simulink model "coupled_tanks_quick_start"  (Simulink 8.3)
settings: Solver=ode1  StartTime=0.0  StopTime=inf  FixedStep=0.1  RelTol=1e-3
PostLoadFcn:
  | qc_set_target_type(getConfigSet(bdroot, 'QUARC Default Target Configuration'));
undefined symbols (not defined in the file or in its folder): HIL
libraries: quarc_library x3
settings Model: Creator=MLevis  LastModifiedBy=Aluno IC  SimulationMode=external  ExtModeTrigDuration=30000
settings SolverCC: PositivePriorityOrder=on
settings OptimizationCC: ExpressionDepthLimit=2147483647  InitFltsAndDblsToZero=on
settings DebuggingCC: SaveWithParameterizedLinksMsg=none  MultiTaskDSMMsg=warning  MultiTaskCondExecSysMsg=none  FcnCallInpInsideContextMsg=UseLocalSettings
settings RTWCC: SystemTargetFile=quarc_win64.tlc  TemplateMakefile=quarc_default_tmf  Description=QUARC Win64 Target  ProcessScript=quarc_win64_make_rtw_hook
settings STFCustomTargetCC: TargetPreCompLibLocation=C:\PROGRA~3\QUARC\lib\2014a\win64\release  ConcurrentExecutionCompliant=on  GeneratePreprocessorConditionals=Disable all  CPPClassGenCompliant=on  SystemTargetFile=quarc_win64.tlc
settings GRTTargetCC: TargetPreCompLibLocation=C:\PROGRA~3\QUARC\lib\2014a\win64\release  ParMdlRefBuildCompliant=off  CompOptLevelCompliant=off  MatFileLogging=off  ExtMode=on  ExtModeMexFile=quarc_comm

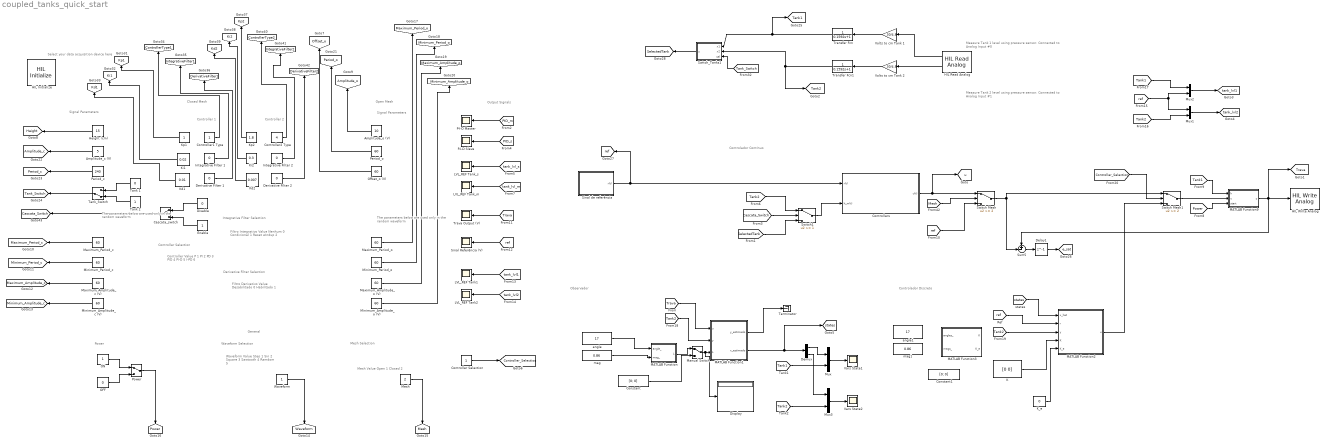
== system coupled_tanks_quick_start ==
  note: Controlador Discreto
  note: Observador
  note: Controlador Contínuo
  note: Measure Tank 2 level using pressure sensor.
      | Connected to Analog Input #1
  note: Measure Tank 1 level using pressure sensor.
      | Connected to Analog Input #0
  note: Select your data acquisition device here
  note: Output Signals
  note: Controller
      | Value
      |
      | P
      | 1
      |
      | PI
      | 2
      |
      | PD
      | 3
      |
      | PID
      | 4
      |
      | PI-D
      | 5
      |
      | I-PD
      | 6
  note: Controller Selection
  note: Signal Parameters
  note: Mesh
      | Value
      |
      | Open
      | 1
      |
      | Closed
      | 2
  note: Mesh Selection
  note: Power
  note: Waveform
      | Value
      |
      | Step
      | 1
      |
      | Sin
      | 2
      |
      | Square
      | 3
      |
      | Sawtooth
      | 4
      |
      | Ramdom
      | 5
  note: Waveform Selection
  note: General
  note: Controller 1
  note: The parameters below are used only in the random waveform
  note: Signal Parameters
  note: The parameters below are used only in the random waveform
  note: Open Mesh
  note: Controller 2
  note: Filtro Derivativo
      | Value
      |
      | Desabilitado
      | 0
      |
      | Habilitado
      | 1
  note: Filtro Integrativo
      | Value
      |
      | Nenhum
      | 0
      |
      | Condicional
      | 1
      |
      | Reset windup
      | 2
  note: Integrative Filter Selection
  note: Derivative Filter Selection
  note: Closed Mesh
  Amplitude_c (V) : Constant  Value=5
  Amplitude_o (V) : Constant  Value=10
  Cascata_switch : ManualSwitch
  Constant : Constant  Value=[0; 0]
  Constant1 : Constant  Value=[0; 0]
  Controller Selection : Constant
  Controller1 Type : Constant
  Controller2 Type : Constant  Value=4
  Controllers : Subsystem
  Delay1 : Delay  DelayLength=1  InitialCondition=0
  Demux : Demux  Outputs=2
  Derivative Filter 1 : Constant  Value=0
  Derivative Filter 2 : Constant  Value=0
  Disable : Constant  Value=0
  Display : Display
  Enable : Constant
  HIL Initialize : quarc_library/Data Acquisition/Generic/Configuration/HIL Initialize  object_name=HIL-1  board_type=q2_usb  board_number=0  board_options=d0=digital;d1=digital;led=auto;update_rate=normal;decimation=1  exclusive=off  active=off  hardware_clocks=[0]  clock_modes=[]  initial_clock_frequencies=[]  set_clock_params_at_start=off  set_clock_params_at_switch_in=off  set_clock_frequencies_at_start=off  set_clock_frequencies_at_switch_in=off  analog_input_channels=[0:1]  analog_input_maximums=10  analog_input_minimums=-10  set_analog_input_params_at_start=on  set_analog_input_params_at_switch_in=off  analog_output_channels=[0:1]  analog_output_maximums=10  analog_output_minimums=-10  initial_analog_outputs=[0]  final_analog_outputs=[0]  watchdog_analog_outputs=0  set_analog_output_params_at_start=on  set_analog_output_params_at_switch_in=off  set_analog_outputs_at_start=on  set_analog_outputs_at_switch_in=off  set_analog_outputs_at_terminate=on  set_analog_outputs_at_switch_out=off  set_analog_outputs_on_watchdog=off  digital_input_channels=[]  digital_output_channels=[]  digital_output_configuration=[]  initial_digital_outputs=[1]  final_digital_outputs=[1]  watchdog_digital_outputs=[1]  set_digital_output_params_at_start=off  set_digital_output_params_at_switch_in=off  set_digital_outputs_at_start=on  set_digital_outputs_at_switch_in=off  set_digital_outputs_at_terminate=on  set_digital_outputs_at_switch_out=off  set_digital_outputs_on_watchdog=off  encoder_channels=[0:1]  quadrature=[4]  encoder_filter_frequency=[]  initial_encoder_counts=[0]  set_encoder_params_at_start=on  set_encoder_params_at_switch_in=off  set_encoder_counts_at_start=on  set_encoder_counts_at_switch_in=off  pwm_channels=[]  pwm_modes=[0]  pwm_frequency=1/0.020  pwm_configuration=[]  pwm_alignment=[]  pwm_polarity=[]  pwm_leading_deadband=[]  pwm_trailing_deadband=[]  initial_pwm_outputs=[0]  final_pwm_outputs=[0]  watchdog_pwm_outputs=[0]  set_pwm_params_at_start=on  set_pwm_params_at_switch_in=off  set_pwm_outputs_at_start=on  set_pwm_outputs_at_switch_in=off  set_pwm_outputs_at_terminate=on  set_pwm_outputs_at_switch_out=off  set_pwm_outputs_on_watchdog=off  other_output_channels=[]  initial_other_outputs=[]  final_other_outputs=[]  watchdog_other_outputs=[]  set_other_outputs_at_start=off  set_other_outputs_at_switch_in=off  set_other_outputs_at_terminate=off  set_other_outputs_at_switch_out=off  set_other_outputs_on_watchdog=off
  HIL Read Analog : quarc_library/Data Acquisition/Generic/Immediate I//O/HIL Read Analog  object_name=HIL-1  channels=[0:1]  sample_time=qc_get_step_size  active=on  vector_output=off
  HIL Write Analog : quarc_library/Data Acquisition/Generic/Immediate I//O/HIL Write Analog  object_name=HIL-1  channels=0  sample_time=-1  active=off  vector_input=off
  Height (cm) : Constant  Value=15
  Integrative Filter 1 : Constant  Value=0
  Integrative Filter 2 : Constant  Value=0
  K : Constant  Value=[0 0]  VectorParams1D=off
  K_e : Constant  Value=0  VectorParams1D=off
  Kd1 : Constant  Value=0.01
  Kd2 : Constant  Value=0.007
  Ki1 : Constant  Value=0.02
  Ki2 : Constant  Value=0.3
  Kp1 : Constant
  Kp2 : Constant  Value=1.8
  LVL_REF Tank1 : Scope
      settings: ShowLegends=on  TimeRange=100  YMin=0  YMax=30  SaveName=tank1level1
  LVL_REF Tank2 : Scope
      settings: ShowLegends=on  TimeRange=250  YMin=0  YMax=30  SaveName=tank2level1
  "LVL_REF Tank_m " : Scope
      settings: ShowLegends=on  TimeRange=300  YMin=0  YMax=30  SaveName=tank2level
  LVL_REF Tank_s : Scope
      settings: ShowLegends=on  TimeRange=300  YMin=-90  YMax=130  SaveName=tank1level
  MATLAB Function : MATLAB Function  TreatAsAtomicUnit=on
  MATLAB Function1 : MATLAB Function  TreatAsAtomicUnit=on
  MATLAB Function2 : MATLAB Function  TreatAsAtomicUnit=on
  MATLAB Function3 : MATLAB Function  TreatAsAtomicUnit=on
  MATLAB Function9 : MATLAB Function  TreatAsAtomicUnit=on
  Manual Switch : ManualSwitch
  Maximum_Amplitude_c (V) : Constant  Value=60
  Maximum_Amplitude_o (V) : Constant  Value=60
  Maximum_Period_c : Constant  Value=60
  Maximum_Period_o : Constant  Value=60
  Mesh : Constant  Value=2
  Minimum_Amplitude_c (V) : Constant  Value=60
  Minimum_Amplitude_o (V) : Constant  Value=60
  Minimum_Period_c : Constant  Value=60
  Minimum_Period_o : Constant  Value=60
  Mux{,1..3} (4 alike) : Mux  Inputs=2
  OFF : Constant  Value=0
  ON : Constant
  Offset_o (V) : Constant  Value=60
  P-I-D Master : Scope
      settings: ShowLegends=on  TimeRange=300  YMin=-35  YMax=30  SaveName=PID1
  P-I-D Slave : Scope
      settings: ShowLegends=on  TimeRange=300  YMin=-35  YMax=80  SaveName=PID2
  Period_c : Constant  Value=240
  Period_o : Constant  Value=60
  Power : ManualSwitch
  Sinal Referência (V) : Scope
      settings: TimeRange=300  YMin=0  YMax=30  SaveName=meshoutput
  Sinal de referência : Subsystem
  Sum5 : Sum  Inputs=+-|
  Switch Mesh : Switch  Threshold=2
  Switch Mesh1 : Switch  Threshold=2
  Switch1 : Switch  Threshold=1
  Switch_Tanks1 : MATLAB Function  TreatAsAtomicUnit=on
  Tank 1 : Constant  Value=0
  Tank 2 : Constant
  Tank_Switch : ManualSwitch  CurrentSetting=0
  Terminator : Terminator
  Transfer Fcn : TransferFcn  Denominator=[0.1592 1]
  Transfer Fcn1 : TransferFcn  Denominator=[0.1592 1]
  Trava Output (V) : Scope
      settings: TimeRange=300  YMin=-4.5  YMax=4.5  SaveName=meshoutput2
  Vars State1 : Scope
      settings: ShowLegends=on  TimeRange=100  YMin=-1  YMax=30  SaveName=state1
  Vars State2 : Scope
      settings: ShowLegends=on  TimeRange=100  YMin=-1  YMax=30  SaveName=state2
  "Volts to cm Tank 1 " : Gain  Gain=30/4.8
  Volts to cm Tank 2 : Gain  Gain=30/4.8
  Waveform : Constant
  angle : Constant  Value=17
  angle1 : Constant  Value=17
  mag : Constant  Value=0.86
  mag1 : Constant  Value=0.86
  tag scope: Amplitude_c=global, Amplitude_o=global, Cascata_Switch=global, ControllerType1=global, ControllerType2=global, Controller_Selection=global, DerivativeFilter1=global, DerivativeFilter2=global, Height=global, IntegrativeFilter1=global, IntegrativeFilter2=global, Kd1=global, Kd2=global, Ki1=global, Ki2=global, Kp1=global, Kp2=global, Maximum_Amplitude_c=global, Maximum_Amplitude_o=global, Maximum_Period_c=global, Maximum_Period_o=global, Mesh=global, Minimum_Amplitude_c=global, Minimum_Amplitude_o=global, Minimum_Period_c=global, Minimum_Period_o=global, Offset_o=global, Period_c=global, Period_o=global, Power=global, SelectedTank=global, Tank1=global, Tank2=global, Tank_Switch=global, Trava=global, Waveform=global, e_sat=global, ref=global, states=global, tank_lvl1=global, tank_lvl2=global, u=global
  wires:
  HIL Read Analog/1 -> "Volts to cm Tank 1 "/1
  "Volts to cm Tank 1 "/1 -> Transfer Fcn/1
  Volts to cm Tank 2/1 -> Transfer Fcn1/1
  HIL Read Analog/2 -> Volts to cm Tank 2/1
  [Cascata_Switch] -> Switch1/2
  [SelectedTank] -> Switch1/3
  [Tank2] -> Switch1/1
  ON/1 -> Power/1
  OFF/1 -> Power/2
  Tank 1/1 -> Tank_Switch/1
  Tank 2/1 -> Tank_Switch/2
  Height (cm)/1 -> [Height]
  Tank_Switch/1 -> [Tank_Switch]
  Amplitude_c (V)/1 -> [Amplitude_c]
  Period_c/1 -> [Period_c]
  Maximum_Period_c/1 -> [Maximum_Period_c]
  Minimum_Period_c/1 -> [Minimum_Period_c]
  Maximum_Amplitude_c (V)/1 -> [Maximum_Amplitude_c]
  Minimum_Amplitude_c (V)/1 -> [Minimum_Amplitude_c]
  Waveform/1 -> [Waveform]
  Mesh/1 -> [Mesh]
  Power/1 -> [Power]
  Amplitude_o (V)/1 -> [Amplitude_o]
  Period_o/1 -> [Period_o]
  Offset_o (V)/1 -> [Offset_o]
  Maximum_Period_o/1 -> [Maximum_Period_o]
  Minimum_Period_o/1 -> [Minimum_Period_o]
  Maximum_Amplitude_o (V)/1 -> [Maximum_Amplitude_o]
  Minimum_Amplitude_o (V)/1 -> [Minimum_Amplitude_o]
  Kp1/1 -> [Kp1]
  Ki1/1 -> [Ki1]
  Kd1/1 -> [Kd1]
  Controller1 Type/1 -> [ControllerType1]
  Integrative Filter 1/1 -> [IntegrativeFilter1]
  Derivative Filter 1/1 -> [DerivativeFilter1]
  Kp2/1 -> [Kp2]
  Ki2/1 -> [Ki2]
  Kd2/1 -> [Kd2]
  Derivative Filter 2/1 -> [DerivativeFilter2]
  Integrative Filter 2/1 -> [IntegrativeFilter2]
  Controller2 Type/1 -> [ControllerType2]
  Disable/1 -> Cascata_switch/1
  Enable/1 -> Cascata_switch/2
  Cascata_switch/1 -> [Cascata_Switch]
  Switch Mesh/1 -> Switch Mesh1/1, Sum5/2
  [Tank1] -> MATLAB Function9/1(h)
  [Mesh] -> Switch Mesh/2
  Switch_Tanks1/1(y) -> [SelectedTank]
  Sinal de referência/1(r(t)) -> Controllers/1(r(t)), [ref]
  [Tank_Switch] -> Switch_Tanks1/3(sel)
  Transfer Fcn1/1 -> Switch_Tanks1/2(x2), [Tank2]
  Transfer Fcn/1 -> Switch_Tanks1/1(x1), [Tank1]
  [Power] -> MATLAB Function9/3(start)
  Controllers/1(u(t)) -> [u], Switch Mesh/1
  MATLAB Function9/1(y) -> [Trava], Sum5/1, HIL Write Analog/1
  Delay1/1 -> [e_sat]
  Sum5/1 -> Delay1/1
  [ref] -> Switch Mesh/3
  Switch1/1 -> Controllers/2(h_m(t))
  [PID_m] -> P-I-D Master/1
  [PID_s] -> P-I-D Slave/1
  [tank_lvl_m] -> "LVL_REF Tank_m "/1
  [tank_lvl_s] -> LVL_REF Tank_s/1
  [Trava] -> Trava Output (V)/1
  [ref] -> Sinal Referência (V)/1
  [Tank1] -> Mux2/1
  [ref] -> Mux2/2, Mux1/1
  [Tank2] -> Mux1/2
  Mux2/1 -> [tank_lvl1]
  Mux1/1 -> [tank_lvl2]
  [tank_lvl1] -> LVL_REF Tank1/1
  [tank_lvl2] -> LVL_REF Tank2/1
  mag/1 -> MATLAB Function/2(mag_)
  angle/1 -> MATLAB Function/1(angle_)
  [Trava] -> MATLAB Function1/1(u)
  [Tank2] -> MATLAB Function1/2(y)
  MATLAB Function1/2(x_estimado) -> [states], Demux/1
  Mux/1 -> Vars State1/1
  [Tank1] -> Mux/2
  Constant/1 -> Manual Switch/2
  Demux/1 -> Mux/1
  Demux/2 -> Mux3/1
  [Tank2] -> Mux3/2
  Mux3/1 -> Vars State2/1
  Manual Switch/1 -> Display/1, MATLAB Function1/3(L)
  MATLAB Function/1(L) -> Manual Switch/1
  MATLAB Function1/1(y_estimado) -> Terminator/1
  [states] -> MATLAB Function2/1(x_hat)
  [ref] -> MATLAB Function2/2(r)
  [Tank2] -> MATLAB Function2/3(y)
  K/1 -> MATLAB Function2/4(K)
  K_e/1 -> MATLAB Function2/5(K_e)
  Switch Mesh1/1 -> MATLAB Function9/2(u)
  MATLAB Function2/1(u) -> Switch Mesh1/3
  [Controller_Selection] -> Switch Mesh1/2
  Controller Selection/1 -> [Controller_Selection]

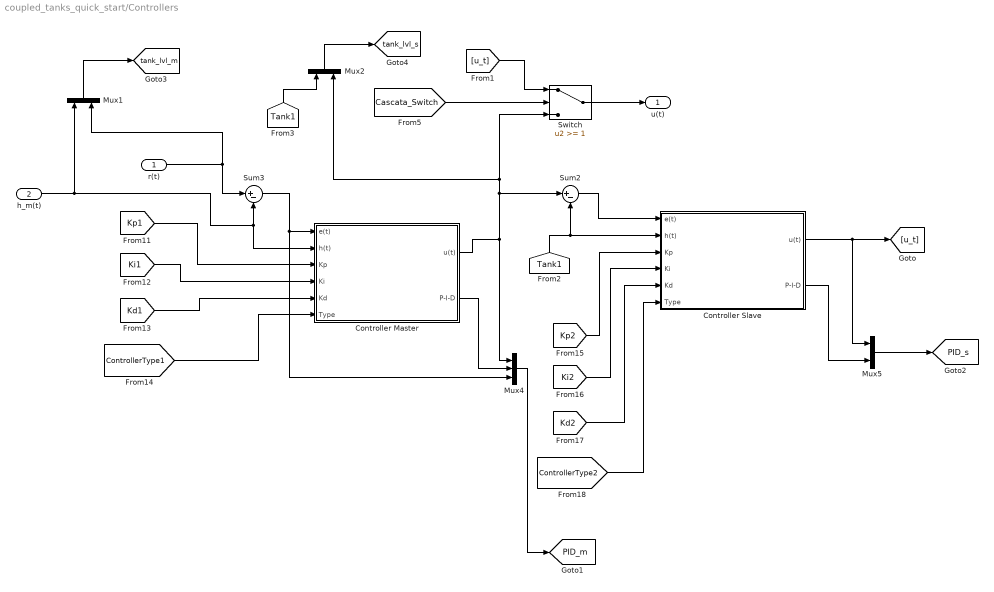
== system coupled_tanks_quick_start/Controllers ==
  r(t) : Inport
  h_m(t) : Inport  Port=2
  Controller Master : Subsystem
  Controller Slave : Subsystem
  Mux1 : Mux  Inputs=2
  Mux2 : Mux  Inputs=2
  Mux4 : Mux  Inputs=3
  Mux5 : Mux  Inputs=2
  Sum2 : Sum  Inputs=|+-
  Sum3 : Sum  Inputs=|+-
  Switch : Switch  Threshold=1
  u(t) : Outport
  tag scope: PID_m=global, PID_s=global, tank_lvl_m=global, tank_lvl_s=global
  wires:
  [Tank1] -> Controller Slave/2(h(t)), Sum2/2
  [Kd1] -> Controller Master/5(Kd)
  Controller Slave/2(P-I-D) -> Mux5/2
  [Kp2] -> Controller Slave/3(Kp)
  [Ki2] -> Controller Slave/4(Ki)
  [Ki1] -> Controller Master/4(Ki)
  [Kd2] -> Controller Slave/5(Kd)
  [ControllerType2] -> Controller Slave/6(Type)
  [Kp1] -> Controller Master/3(Kp)
  [ControllerType1] -> Controller Master/6(Type)
  h_m(t)/1 -> Sum3/2, Controller Master/2(h(t)), Mux1/1
  Controller Master/1(u(t)) -> Mux2/2, Switch/3, Sum2/1, Mux4/1
  Sum2/1 -> Controller Slave/1(e(t))
  Controller Slave/1(u(t)) -> [u_t], Mux5/1
  r(t)/1 -> Sum3/1, Mux1/2
  Switch/1 -> u(t)/1
  [Cascata_Switch] -> Switch/2
  Sum3/1 -> Mux4/3, Controller Master/1(e(t))
  [u_t] -> Switch/1
  Mux1/1 -> [tank_lvl_m]
  [Tank1] -> Mux2/1
  Mux2/1 -> [tank_lvl_s]
  Mux4/1 -> [PID_m]
  Mux5/1 -> [PID_s]
  Controller Master/2(P-I-D) -> Mux4/2

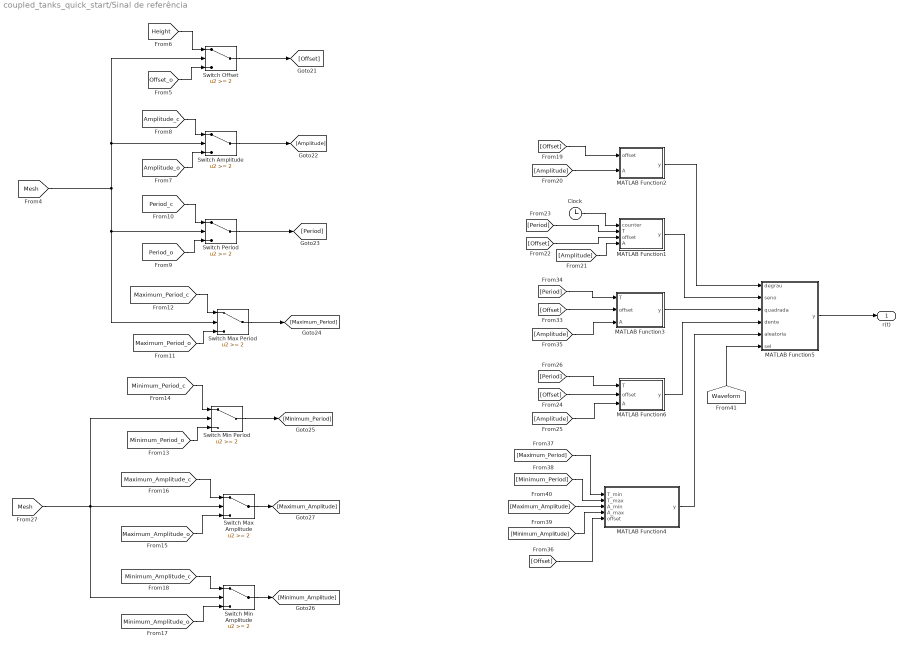
== system coupled_tanks_quick_start/Sinal de referência ==
  Clock : Clock
  MATLAB Function1 : MATLAB Function  TreatAsAtomicUnit=on
  MATLAB Function2 : MATLAB Function  TreatAsAtomicUnit=on
  MATLAB Function3 : MATLAB Function  TreatAsAtomicUnit=on
  MATLAB Function4 : MATLAB Function  TreatAsAtomicUnit=on
  MATLAB Function5 : MATLAB Function  TreatAsAtomicUnit=on
  MATLAB Function6 : MATLAB Function  TreatAsAtomicUnit=on
  Switch Amplitude : Switch  Threshold=2
  Switch Max Amplitude : Switch  Threshold=2
  Switch Max Period : Switch  Threshold=2
  Switch Min Amplitude : Switch  Threshold=2
  Switch Min Period : Switch  Threshold=2
  Switch Offset : Switch  Threshold=2
  Switch Period : Switch  Threshold=2
  r(t) : Outport
  wires:
  Clock/1 -> MATLAB Function1/1(counter)
  MATLAB Function5/1(y) -> r(t)/1
  [Mesh] -> Switch Max Period/2, Switch Period/2, Switch Offset/2, Switch Amplitude/2
  [Offset] -> MATLAB Function6/2(offset)
  Switch Min Amplitude/1 -> [Minimum_Amplitude]
  [Period] -> MATLAB Function6/1(T)
  Switch Amplitude/1 -> [Amplitude]
  Switch Period/1 -> [Period]
  Switch Offset/1 -> [Offset]
  [Amplitude] -> MATLAB Function2/2(A)
  Switch Min Period/1 -> [Minimum_Period]
  [Amplitude] -> MATLAB Function1/4(A)
  Switch Max Amplitude/1 -> [Maximum_Amplitude]
  Switch Max Period/1 -> [Maximum_Period]
  [Offset] -> MATLAB Function1/3(offset)
  [Offset] -> MATLAB Function2/1(offset)
  [Period] -> MATLAB Function1/2(T)
  [Amplitude] -> MATLAB Function6/3(A)
  [Period] -> MATLAB Function3/1(T)
  MATLAB Function1/1(y) -> MATLAB Function5/2(seno)
  [Waveform] -> MATLAB Function5/6(sel)
  [Maximum_Period] -> MATLAB Function4/1(T_min)
  [Mesh] -> Switch Min Amplitude/2, Switch Max Amplitude/2, Switch Min Period/2
  MATLAB Function2/1(y) -> MATLAB Function5/1(degrau)
  [Maximum_Amplitude] -> MATLAB Function4/3(A_min)
  MATLAB Function6/1(y) -> MATLAB Function5/4(dente)
  [Amplitude] -> MATLAB Function3/3(A)
  [Minimum_Amplitude] -> MATLAB Function4/4(A_max)
  [Offset] -> MATLAB Function4/5(offset)
  MATLAB Function4/1(y) -> MATLAB Function5/5(aleatoria)
  MATLAB Function3/1(y) -> MATLAB Function5/3(quadrada)
  [Offset] -> MATLAB Function3/2(offset)
  [Minimum_Period] -> MATLAB Function4/2(T_max)
  [Offset_o] -> Switch Offset/3
  [Height] -> Switch Offset/1
  [Amplitude_o] -> Switch Amplitude/3
  [Amplitude_c] -> Switch Amplitude/1
  [Period_o] -> Switch Period/3
  [Period_c] -> Switch Period/1
  [Maximum_Period_o] -> Switch Max Period/3
  [Maximum_Period_c] -> Switch Max Period/1
  [Minimum_Period_c] -> Switch Min Period/1
  [Minimum_Period_o] -> Switch Min Period/3
  [Maximum_Amplitude_c] -> Switch Max Amplitude/1
  [Maximum_Amplitude_o] -> Switch Max Amplitude/3
  [Minimum_Amplitude_c] -> Switch Min Amplitude/1
  [Minimum_Amplitude_o] -> Switch Min Amplitude/3

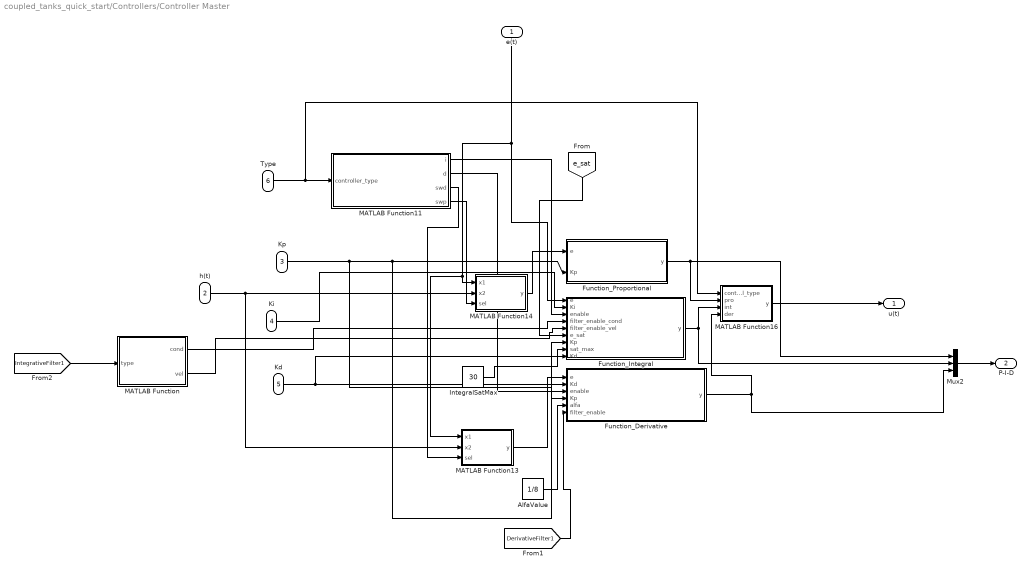
== system coupled_tanks_quick_start/Controllers/Controller Master ==
  e(t) : Inport
  h(t) : Inport  Port=2
  Kp : Inport  Port=3
  Ki : Inport  Port=4
  Kd : Inport  Port=5
  Type : Inport  Port=6
  AlfaValue : Constant  Value=1/8
  Function_Derivative : MATLAB Function  TreatAsAtomicUnit=on
  Function_Integral : MATLAB Function  TreatAsAtomicUnit=on
  Function_Proportional : MATLAB Function  TreatAsAtomicUnit=on
  IntegralSatMax : Constant  Value=30
  MATLAB Function : MATLAB Function  TreatAsAtomicUnit=on
  MATLAB Function11 : MATLAB Function  TreatAsAtomicUnit=on
  MATLAB Function13 : MATLAB Function  TreatAsAtomicUnit=on
  MATLAB Function14 : MATLAB Function  TreatAsAtomicUnit=on
  MATLAB Function16 : MATLAB Function  TreatAsAtomicUnit=on
  Mux2 : Mux  Inputs=3
  u(t) : Outport
  P-I-D : Outport  Port=2
  wires:
  h(t)/1 -> MATLAB Function13/2(x2), MATLAB Function14/2(x2)
  e(t)/1 -> MATLAB Function13/1(x1), MATLAB Function14/1(x1), Function_Integral/1(e)
  Function_Integral/1(y) -> MATLAB Function16/3(int), Mux2/2
  Kp/1 -> Function_Derivative/4(Kp), Function_Integral/7(Kp), Function_Proportional/2(Kp)
  MATLAB Function11/2(d) -> Function_Derivative/3(enable)
  Function_Proportional/1(y) -> MATLAB Function16/2(pro), Mux2/1
  MATLAB Function11/1(i) -> Function_Integral/3(enable)
  Type/1 -> MATLAB Function16/1(control_type), MATLAB Function11/1(controller_type)
  MATLAB Function11/4(swp) -> MATLAB Function14/3(sel)
  Ki/1 -> Function_Integral/2(Ki)
  MATLAB Function/2(vel) -> Function_Integral/5(filter_enable_vel)
  MATLAB Function11/3(swd) -> MATLAB Function13/3(sel)
  MATLAB Function/1(cond) -> Function_Integral/4(filter_enable_cond)
  IntegralSatMax/1 -> Function_Integral/8(sat_max)
  MATLAB Function14/1(y) -> Function_Proportional/1(e)
  AlfaValue/1 -> Function_Derivative/5(alfa)
  [DerivativeFilter1] -> Function_Derivative/6(filter_enable)
  Function_Derivative/1(y) -> MATLAB Function16/4(der), Mux2/3
  MATLAB Function13/1(y) -> Function_Derivative/1(e)
  Kd/1 -> Function_Integral/9(Kd), Function_Derivative/2(Kd)
  Mux2/1 -> P-I-D/1
  MATLAB Function16/1(y) -> u(t)/1
  [e_sat] -> Function_Integral/6(e_sat)
  [IntegrativeFilter1] -> MATLAB Function/1(type)

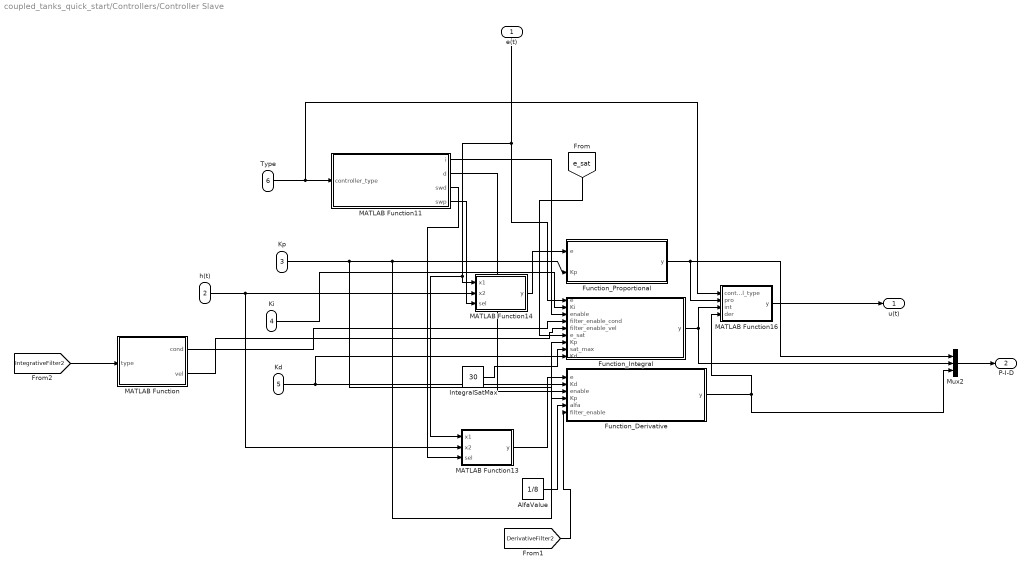
== system coupled_tanks_quick_start/Controllers/Controller Slave ==
  e(t) : Inport
  h(t) : Inport  Port=2
  Kp : Inport  Port=3
  Ki : Inport  Port=4
  Kd : Inport  Port=5
  Type : Inport  Port=6
  AlfaValue : Constant  Value=1/8
  Function_Derivative : MATLAB Function  TreatAsAtomicUnit=on
  Function_Integral : MATLAB Function  TreatAsAtomicUnit=on
  Function_Proportional : MATLAB Function  TreatAsAtomicUnit=on
  IntegralSatMax : Constant  Value=30
  MATLAB Function : MATLAB Function  TreatAsAtomicUnit=on
  MATLAB Function11 : MATLAB Function  TreatAsAtomicUnit=on
  MATLAB Function13 : MATLAB Function  TreatAsAtomicUnit=on
  MATLAB Function14 : MATLAB Function  TreatAsAtomicUnit=on
  MATLAB Function16 : MATLAB Function  TreatAsAtomicUnit=on
  Mux2 : Mux  Inputs=3
  u(t) : Outport
  P-I-D : Outport  Port=2
  wires:
  h(t)/1 -> MATLAB Function13/2(x2), MATLAB Function14/2(x2)
  e(t)/1 -> MATLAB Function13/1(x1), MATLAB Function14/1(x1), Function_Integral/1(e)
  Function_Integral/1(y) -> MATLAB Function16/3(int), Mux2/2
  Kp/1 -> Function_Derivative/4(Kp), Function_Integral/7(Kp), Function_Proportional/2(Kp)
  MATLAB Function11/2(d) -> Function_Derivative/3(enable)
  Function_Proportional/1(y) -> MATLAB Function16/2(pro), Mux2/1
  MATLAB Function11/1(i) -> Function_Integral/3(enable)
  Type/1 -> MATLAB Function16/1(control_type), MATLAB Function11/1(controller_type)
  MATLAB Function11/4(swp) -> MATLAB Function14/3(sel)
  Ki/1 -> Function_Integral/2(Ki)
  MATLAB Function/2(vel) -> Function_Integral/5(filter_enable_vel)
  MATLAB Function11/3(swd) -> MATLAB Function13/3(sel)
  MATLAB Function/1(cond) -> Function_Integral/4(filter_enable_cond)
  IntegralSatMax/1 -> Function_Integral/8(sat_max)
  MATLAB Function14/1(y) -> Function_Proportional/1(e)
  AlfaValue/1 -> Function_Derivative/5(alfa)
  [DerivativeFilter2] -> Function_Derivative/6(filter_enable)
  Function_Derivative/1(y) -> MATLAB Function16/4(der), Mux2/3
  MATLAB Function13/1(y) -> Function_Derivative/1(e)
  Kd/1 -> Function_Integral/9(Kd), Function_Derivative/2(Kd)
  Mux2/1 -> P-I-D/1
  MATLAB Function16/1(y) -> u(t)/1
  [e_sat] -> Function_Integral/6(e_sat)
  [IntegrativeFilter2] -> MATLAB Function/1(type)

== matlab function Controllers/Controller Slave/Function_Derivative ==
  data: e input double; y output double; Kd input double; enable input double; Kp input double; alfa input double; filter_enable input double
function y = derivative(e, Kd, enable, Kp, alfa, filter_enable)

persistent prev_error;
persistent y_error;
persistent aux;

if isempty(prev_error)
   prev_error = 0; 
end

if isempty(y_error)
   y_error = 0; 
end

if isempty(aux)
   aux = 0; 
end


%1/0.1 == 10
Td = Kd/Kp;


if(filter_enable == 1)
    y = ((e - prev_error + alfa*y_error) * Kd)/(1+(Td*alfa));
else
    y = Kd*(e - prev_error)*enable/0.1;
end


prev_error = e;
y_error = y;

end

== matlab function Controllers/Controller Master/MATLAB Function ==
  data: type input double; cond output double; vel output double
function [cond, vel] = IntSwitch(type)

if type == 0
   cond = 0;
   vel = 0;
elseif type == 1
    cond = 1;
    vel = 0;
else
   cond = 0;
   vel = 1;
end

== matlab function Controllers/Controller Slave/Function_Integral ==
  data: e input double; y output double; Ki input double; enable input double; filter_enable_cond input double; filter_enable_vel input double; e_sat input double; Kp input double; sat_max input double; Kd input double
function y = integral(e, Ki, enable, filter_enable_cond, filter_enable_vel, e_sat, Kp, sat_max, Kd)

persistent sum;

if isempty(sum)
   sum = 0; 
end

Ti = Kp/Ki;
Td = Kd/Kp;

Tt = sqrt(Ti * Td);

Tt_value = (1/Tt) * e_sat;

if(filter_enable_cond == 1 && sum > sat_max) 
    sum = 0;
elseif(filter_enable_vel == 1)
    sum =  ((Ki*e) + Tt_value)*0.1 + sum;
else
    sum = sum + Ki*e*0.1;
end
y = sum*enable;

== matlab function Controllers/Controller Slave/Function_Proportional ==
  data: e input double; y output double; Kp input double
function y = proportional(e, Kp)

y = Kp*e;

== matlab function Controllers/Controller Slave/MATLAB Function ==
  data: type input double; cond output double; vel output double
function [cond, vel] = IntSwitch(type)

if type == 0
   cond = 0;
   vel = 0;
elseif type == 1
    cond = 1;
    vel = 0;
else
   cond = 0;
   vel = 1;
end

== matlab function Controllers/Controller Slave/MATLAB Function11 ==
  data: controller_type input double; i output double; d output double; swd output double; swp output double
function [i,d,swd,swp]= fcn(controller_type)

if(controller_type == 1)
    i = 0;
    d = 0;
    swd = 0;
    swp = 0;
elseif(controller_type == 2)
    i = 1;
    d = 0;
    swd = 0;
    swp = 0;
elseif(controller_type == 3)
    i = 0;
    d = 1;
    swd = 0;
    swp = 0;
elseif(controller_type == 4)
    i = 1;
    d = 1;
    swd = 0;
    swp = 0;
elseif(controller_type == 5)
    i = 1;
    d = 1;
    swd = 1;
    swp = 0;
elseif(controller_type == 6)
    i = 1;
    d = 1;
    swd = 1;
    swp = 1;
else
    i = 0;
    d = 0;
    swd = 0;
    swp = 0;
end

== matlab function Controllers/Controller Slave/MATLAB Function13 ==
  data: x1 input double; x2 input double; y output double; sel input double
function y = switch_deriv(x1, x2, sel)

if sel == 0
    y = x1; 
else
    y = x2;
end
    
end

== matlab function Controllers/Controller Master/Function_Proportional ==
  data: e input double; y output double; Kp input double
function y = proportional(e, Kp)

y = Kp*e;

== matlab function Controllers/Controller Slave/MATLAB Function14 ==
  data: x1 input double; x2 input double; y output double; sel input double
function y = switch_prop(x1, x2, sel)

if sel == 0
    y = x1; 
else
    y = x2;
end
    
end

== matlab function Controllers/Controller Master/Function_Integral ==
  data: e input double; y output double; Ki input double; enable input double; filter_enable_cond input double; filter_enable_vel input double; e_sat input double; Kp input double; sat_max input double; Kd input double
function y = integral(e, Ki, enable, filter_enable_cond, filter_enable_vel, e_sat, Kp, sat_max, Kd)

persistent sum;

if isempty(sum)
   sum = 0; 
end

Ti = Kp/Ki;
Td = Kd/Kp;

Tt = sqrt(Ti * Td);

Tt_value = (1/Tt) * e_sat;

if(filter_enable_cond == 1 && sum > sat_max) 
    sum = 0;
elseif(filter_enable_vel == 1)
    sum =  ((Ki*e) + Tt_value)*0.1 + sum;
else
    sum = sum + Ki*e*0.1;
end
y = sum*enable;

== matlab function Controllers/Controller Master/Function_Derivative ==
  data: e input double; y output double; Kd input double; enable input double; Kp input double; alfa input double; filter_enable input double
function y = derivative(e, Kd, enable, Kp, alfa, filter_enable)

persistent prev_error;
persistent y_error;
persistent aux;

if isempty(prev_error)
   prev_error = 0; 
end

if isempty(y_error)
   y_error = 0; 
end

if isempty(aux)
   aux = 0; 
end


%1/0.1 == 10
Td = Kd/Kp;


if(filter_enable == 1)
    y = ((e - prev_error + alfa*y_error)*enable * Kd)/(1+(Td*alfa));
else
    y = Kd*(e - prev_error)*enable/0.1;
end


prev_error = e;
y_error = y;

end

== matlab function Controllers/Controller Master/MATLAB Function11 ==
  data: controller_type input double; i output double; d output double; swd output double; swp output double
function [i,d,swd,swp]= fcn(controller_type)

if(controller_type == 1)
    i = 0;
    d = 0;
    swd = 0;
    swp = 0;
elseif(controller_type == 2)
    i = 1;
    d = 0;
    swd = 0;
    swp = 0;
elseif(controller_type == 3)
    i = 0;
    d = 1;
    swd = 0;
    swp = 0;
elseif(controller_type == 4)
    i = 1;
    d = 1;
    swd = 0;
    swp = 0;
elseif(controller_type == 5)
    i = 1;
    d = 1;
    swd = 1;
    swp = 0;
elseif(controller_type == 6)
    i = 1;
    d = 1;
    swd = 1;
    swp = 1;
else
    i = 0;
    d = 0;
    swd = 0;
    swp = 0;
end

== matlab function MATLAB Function9 ==
  data: h input double; u input double; y output double; start input double
    function y = travas(h, u, start)
%#codegen
h_max = 30;

%Trava de tensÃ£o
if(u < -4)
    u = -4;
end
if(u > 4)
    u = 4;
end

%Trava pra nÃ£o sugar ar
if(u < 0 & h < 2)
    u = 0;
end

%Trava de transbordamento
% if(h >= h_max - 1.0 & h < h_max - 0.75)
%    u = 0.95*u;
% elseif(h >= h_max - 0.75 & h < h_max - 0.5)
%     u = 0.93*u;
% elseif(h >= h_max - 0.5 & h < h_max - 0.25)
%     u = 0.91*u;
% elseif(h >= h_max - 0.25 & h < h_max)
%     u = 0.88*u;
% elseif(h >= h_max)
%     u = 0;
% end

%
if h >= (h_max-1)
    u = (h_max - h)*u;
end

%
% persistent goingup
% 
% if isempty(goingup)
%    goingup = 1; 
% end
% 
% if goingup == 1
%    if h >= 29
%       u = 0;
%       goingup = 0;
%    end
% else
%     if h <= 25
%        goingup = 1; 
%     else
%        u = 0; 
%     end
% end
    
y = start*u;

== matlab function Controllers/Controller Master/MATLAB Function13 ==
  data: x1 input double; x2 input double; y output double; sel input double
function y = switch_deriv(x1, x2, sel)

if sel == 0
    y = x1; 
else
    y = x2;
end
    
end

== matlab function Controllers/Controller Master/MATLAB Function14 ==
  data: x1 input double; x2 input double; y output double; sel input double
function y = switch_prop(x1, x2, sel)

if sel == 0
    y = x1; 
else
    y = x2;
end
    
end

== matlab function Controllers/Controller Slave/MATLAB Function16 ==
  data: control_type input double; y output double; pro input double; int input double; der input double
function y = adding(control_type, pro, int, der)
%#codegen

if(control_type >= 1 && control_type <= 4)
   y = pro + int + der;
elseif(control_type == 5)
    y = pro + int - der;
else
    y = int - pro - der;
end

== matlab function Controllers/Controller Master/MATLAB Function16 ==
  data: control_type input double; y output double; pro input double; int input double; der input double
function y = adding(control_type, pro, int, der)
%#codegen

if(control_type >= 1 && control_type <= 4)
   y = pro + int + der;
elseif(control_type == 5)
    y = pro + int - der;
else
    y = int - pro - der;
end

== matlab function MATLAB Function ==
  data: angle_ input double; L output double; mag_ input double
function L = calc_L(angle_, mag_)

G = [0.9942 0; 0.0057 0.9942];
C = [0 1];

Wo = [C; C*G];

angle_ = angle_*(pi/180);

p1 = complex(pol2cart(angle_, mag_));
p2 = complex(pol2cart(-angle_, mag_));

a1 = real(-(p1+p2));
a2 = real(p1*p2);

qc = G^2 + a1*G + a2*eye(2);
invWo = inv(Wo);
L = qc*invWo*[0; 1];

end

== matlab function MATLAB Function1 ==
  data: u input double; y input double; L input double; y_estimado output double; x_estimado output double
function [y_estimado, x_estimado] = observer(u, y, L)

G = [0.9942 0; 0.0057 0.9942];
H = [0.0739; 0.0002];
C = [0 1];

persistent x_next

if(isempty(x_next))
    x_next = [0; y];
end

x_estimado = x_next;
y_estimado = C*x_estimado;
x_next = G*x_estimado + L*(y-y_estimado) + H*u;

% persistent x_old
% persistent y_old
% 
% if(isempty(x_old))
%     x_old = [0; 0];
% end
% 
% if isempty(y_old)
%    y_old = 0; 
% end
% 
% x_estimado = G*x_old + H*u + L(y-y_old);
% y_estimado = C*x_old;
% 
% x_old = x_estimado;
% y_old = y;

end

== matlab function MATLAB Function2 ==
  data: x_hat input double; r input double; u output double; y input double; K input double; K_e input double
function u = controller(x_hat, r, y, K, K_e)

persistent y_old
persistent r_old

if(isempty(y_old))
    y_old = 0;
    r_old = 0;
end

error = y_old - r_old;
u = -K*x_hat + K_e*error;

y_old = y;
r_old = r;

end

== matlab function MATLAB Function3 ==
  data: angles_ input double; K output double; mags_ input double; K_e output double
function [K, K_e] = calc_K(angles_, mags_)

G = [0.9942 0; 0.0057 0.9942];
H = [0.0739; 0.0002];

Wc = [H; G*H];

angles_ = angles_*(pi/180);

p1 = complex(pol2cart(angles_(1), mags_(1)));
p2 = complex(pol2cart(angles_(2), mags_(2)));
p3 = complex(pol2cart(angles_(3), mags_(3)));

a1 = real(-(p1+p2));
a2 = real(p1*p2);

qc = G^2 + a1*G + a2*eye(2);
invWc = inv(Wc);
K = [0 1]*invWc*qc;



end

== matlab function Sinal de referência/MATLAB Function1 ==
  data: counter input double; y output double; T input double; offset input double; A input double
function y = seno(counter, T, offset, A)

%counter = cast(counter, 'double');

y = A*sin(counter*2*pi/T) + offset;

== matlab function Sinal de referência/MATLAB Function2 ==
  data: offset input double; y output double; A input double
function y = degrau(offset, A)

y = offset;

== matlab function Sinal de referência/MATLAB Function3 ==
  data: y output double; T input double; offset input double; A input double
function y = quadrada(T, offset, A)

persistent counter_q;

if isempty(counter_q)
   counter_q = 0; 
end

counter_q = counter_q + 1;

if (counter_q <= 5*T)
    y = -A + offset;
elseif (counter_q > 5*T)
    y = A + offset;
else
    y = 0;
end

if (counter_q >= 10*T)
   counter_q = 0; 
end

== matlab function Sinal de referência/MATLAB Function4 ==
  data: T_min input double; y output double; T_max input double; A_min input double; A_max input double; offset input double
function y = aleatoria(T_min, T_max, A_min, A_max, offset)

persistent T_now;
persistent A_now;
persistent counter_a;

if isempty(counter_a)
    T_now = T_min + (T_max - T_min)*rand;
    A_now = A_min + (A_max - A_min)*rand + offset;
    counter_a = 0;
end

counter_a = counter_a + 1;

y = A_now;

if (counter_a >= T_now*10)
    T_now = T_min + (T_max - T_min)*rand;
    A_now = A_min + (A_max - A_min)*rand + offset;
    counter_a = 0;
end

== matlab function Sinal de referência/MATLAB Function5 ==
  data: degrau input double; y output double; seno input double; quadrada input double; dente input double; aleatoria input double; sel input double
function y = mux(degrau, seno, quadrada, dente, aleatoria, sel)

switch sel
    case 1
        y = degrau;
    case 2
        y = seno;
    case 3
        y = quadrada;
    case 4
        y = dente;
    case 5
        y = aleatoria;
    otherwise
        y = 0;
end

== matlab function Sinal de referência/MATLAB Function6 ==
  data: y output double; T input double; offset input double; A input double
function y = dente(T, offset, A)

persistent counter_d;

if isempty(counter_d)
   counter_d = 0; 
end


y = counter_d*A*2/(10*T) + offset - A;

counter_d = counter_d + 1;

if (counter_d > T*10)
   counter_d = 0;
end

== matlab function Switch_Tanks1 ==
  data: x1 input double; x2 input double; y output double; sel input double
function y = switch2(x1, x2, sel)

if sel == 0
    y = x1; 
else
    y = x2;
end
    
end
